simulink model "simula_gpc_generic_dU"  (R2018a)
settings: Solver=VariableStepAuto  StartTime=0.0  StopTime=Tsim  RelTol=1e-3
values from neighbouring files (symbols this model uses):
  delta = [1 -1]    [gpc_generic_dU.m]
  GPC = gpc_tf2ss_dU(Pz,[],delta,3,3)    [gpc_generic_dU.m]
  Qd = 1*eye(GPC.n*GPC.nout)    [gpc_generic_dU.m]
  Ql = lambda*eye(GPC.nu*GPC.nin)    [gpc_generic_dU.m]
  Ts = 1    [gpc_generic_dU.m]
  Tsim = 12    [gpc_generic_dU.m]
libraries: simulink x1, cstblocks x1
settings Model: Creator=marcus  LastModifiedBy=marcus

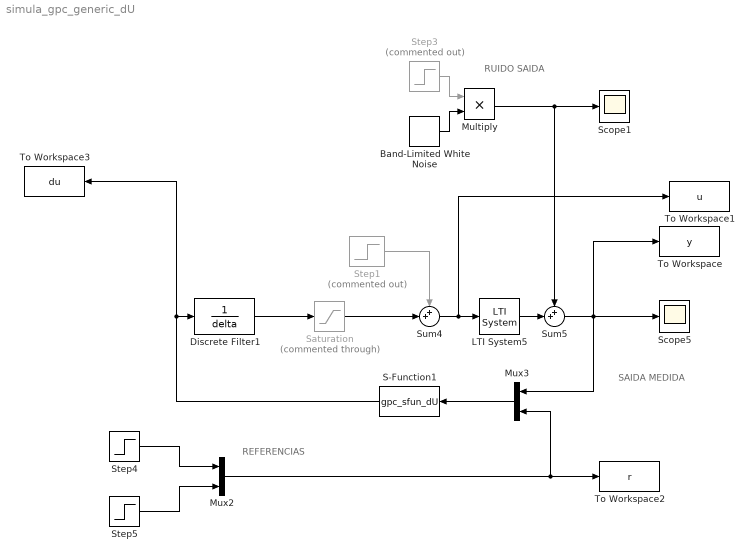
== system simula_gpc_generic_dU ==
  note: SAIDA MEDIDA
  note: REFERENCIAS
  note: RUIDO SAIDA
  Band-Limited White Noise : simulink/Sources/Band-Limited White Noise  Cov=Ts/5000  Ts=Ts/10  seed=[23341]
  Discrete Filter1 : DiscreteFilter  Numerator=1  Denominator=delta  SampleTime=Ts
  LTI System5 : cstblocks/LTI System  sys=P  IC=[]
  Multiply : Product
  Mux2 : Mux  Inputs=2
  Mux3 : Mux  Inputs=2
  S-Function1 : S-Function  FunctionName=gpc_sfun_dU  Parameters=GPC,Ql,Qd  SFunctionDeploymentMode=off  EnableBusSupport=off
  Saturation : Saturate  Commented=through  UpperLimit=0.4  LowerLimit=0
  Scope1 : Scope
  Scope5 : Scope
  Step1 : Step  Commented=on  Time=Tsim/2  SampleTime=0
  Step3 : Step  Commented=on  Time=4*Tsim/5  SampleTime=0
  Step4 : Step  Time=0  SampleTime=Ts
  Step5 : Step  Time=Tsim/2  After=0.5  SampleTime=Ts
  Sum4 : Sum  Inputs=++|
  Sum5 : Sum  Inputs=++|
  To Workspace : ToWorkspace  VariableName=y  SaveFormat=Timeseries  SampleTime=Ts
  To Workspace1 : ToWorkspace  VariableName=u  SaveFormat=Timeseries  SampleTime=Ts
  To Workspace2 : ToWorkspace  VariableName=r  SaveFormat=Timeseries  SampleTime=-1
  To Workspace3 : ToWorkspace  VariableName=du  SaveFormat=Timeseries  SampleTime=Ts
  wires:
  Mux2/1 -> Mux3/2, To Workspace2/1
  Mux3/1 -> S-Function1/1
  Sum4/1 -> To Workspace1/1, LTI System5/1
  Discrete Filter1/1 -> Saturation/1
  Step1/1 -> Sum4/1
  Step3/1 -> Multiply/1
  Multiply/1 -> Sum5/1, Scope1/1
  Band-Limited White Noise/1 -> Multiply/2
  LTI System5/1 -> Sum5/2
  Sum5/1 -> To Workspace/1, Mux3/1, Scope5/1
  S-Function1/1 -> To Workspace3/1, Discrete Filter1/1
  Step5/1 -> Mux2/2
  Step4/1 -> Mux2/1
  Saturation/1 -> Sum4/2
